simulink model "KD_cl_harness_forthao_breach"  (R2015a)
settings: Solver=ode45  StartTime=0  StopTime=50  FixedStep=0.01  MaxStep=0.005  RelTol=1e-4  AbsTol=1e-4
InitFcn:
  | load KD_const_coeffs_0624
  | load pexhat_stuff
  | load expcon
  | load thr_ff_map
undefined symbols (not defined in the file): c_0, c_1, c_100, c_1000, c_10000, c_1000inv, c_100inv, c_1_int, c_1d2p4, c_1p7, c_4400inv, c_5500inv, c_80, c_90, c_cal_phi, c_compmap, c_ctok, c_fflow_max, c_fflow_min, c_filt, c_flowdiv, c_flowmin, c_flowmult, c_inf, c_km1d2k, c_mm3tokgpers, c_n1, c_p00001, c_p01, c_p016, c_p1429, c_p1e9, c_p4167, c_p4d1p4, c_p5401, c_p9, c_pincomp, c_ra, c_rair, c_Rby1000, c_roacorr, c_rpmtoradpers, c_svrthrottle1, c_svrthrottle2, c_svrthrottlearg, c_svrthrottlebeta, c_ta_max, c_ta_min, c_V, c_vnliftmax, c_vnliftmin, Coefs, const, const_exhat, eegr_map, egrr_delay_init, epim_map, eplufin_ff_map, expcon, invta ... (+17)
libraries: simulink x5
(part 3 of 5)

== system KD_cl_harness_forthao_breach/ctrl_rb_explicit_20131031_v2/While_Iterator_Subsystem ==
  In1 : Inport
  In2 : Inport  Port=2
  In3 : Inport  Port=3
  In4 : Inport  Port=4
  In5 : Inport  Port=5
  In6 : Inport  Port=6
  In7 : Inport  Port=7
  In8 : Inport  Port=8
  pexz : Inport  Port=9
  Constant10 : Constant  Value=SVR_EGR_exhat.Beta
  Constant11 : Constant  Value=SVR_EGR_exhat.SV2
  Constant12 : Constant  Value=SVR_EGR_exhat.SV1
  Constant13 : Constant  Value=const_exhat.k
  Constant14 : Constant  Value=SVR_EGR_exhat.arg
  Constant7 : Constant  Value=const_exhat.Pcab
  Constant8 : Constant  Value=const_exhat.Tcab
  Gain10 : Gain  Gain=c_p01
      settings: AttributesFormatString=%<Gain>
  Gain11 : Gain  Gain=c_4400inv
      settings: AttributesFormatString=%<Gain>
  Mux14 : Mux  Inputs=2
  Saturation4 : Saturate  UpperLimit=c_inf  LowerLimit=c_80
      settings: AttributesFormatString=%<LowerLimit>\n%<UpperLimit>
  Saturation_Dynamic2 : simulink/Discontinuities/Saturation Dynamic  OutMin=[]  OutMax=[]  OutDataTypeStr=Inherit: Same as second input  OutDataType=fixdt(1, 16)  OutScaling=2^-10  DoSatur=off
  Sum14 : Sum  Inputs=++|
  While Iterator : WhileIterator
  newton : Subsystem
  pexmax1 : Constant  Value=1000  OutDataTypeStr=single  SampleTime=-1
      settings: AttributesFormatString=%<Value>\n%<SampleTime>
  unity2 : Constant  OutDataTypeStr=single  SampleTime=-1
      settings: AttributesFormatString=%<Value>\n%<SampleTime>
  y_cons4 : Constant  OutDataTypeStr=boolean  SampleTime=-1
      settings: AttributesFormatString=%<Value>\n%<SampleTime>
  Out1 : Outport
  Out2 : Outport  Port=2
  Out3 : Outport  Port=3
  wires:
  y_cons4/1 -> While Iterator/1
  Constant14/1 -> newton/5(arg)
  Constant12/1 -> newton/3(SV1)
  Constant10/1 -> newton/2(Beta)
  Gain11/1 -> Mux14/2
  Gain10/1 -> Mux14/1
  Mux14/1 -> newton/1(u)
  Constant7/1 -> newton/9(pcab)
  Constant8/1 -> newton/10(tcab)
  Constant13/1 -> newton/12(k)
  newton/1(pexkp1) -> Out1/1, Saturation_Dynamic2/2
  Saturation_Dynamic2/1 -> Out3/1
  unity2/1 -> Sum14/1
  Sum14/1 -> Saturation_Dynamic2/3
  pexmax1/1 -> Saturation_Dynamic2/1
  Constant11/1 -> newton/4(SV2)
  Saturation4/1 -> Sum14/2
  In1/1 -> Gain10/1
  In2/1 -> Gain11/1
  In3/1 -> newton/7(pin)
  In4/1 -> newton/8(wegrmeas)
  newton/2(dwdp) -> Out2/1
  In5/1 -> newton/11(tex)
  In6/1 -> newton/13(pex_ecu)
  In7/1 -> Saturation4/1
  In8/1 -> While Iterator/2
  pexz/1 -> newton/6(pex)

== system KD_cl_harness_forthao_breach/ctrl_rb_explicit_20131031_v2/custom_filter ==
  Input : Inport
  Data Store Read1 : DataStoreRead  DataStoreName=man_tuneFiltalpha  SampleTime=sample_time
  Data Store Read8 : DataStoreRead  DataStoreName=man_tuneFiltalpha  SampleTime=sample_time
  Delay1 : Delay  DelayLength=1  InitialCondition=0
  Product1 : Product  Inputs=**  RndMeth=Zero
  Product2 : Product  Inputs=**  RndMeth=Zero
  Saturation1 : Saturate  UpperLimit=1  LowerLimit=0
      settings: AttributesFormatString=%<LowerLimit>\n%<UpperLimit>
  Saturation4 : Saturate  UpperLimit=1  LowerLimit=0
      settings: AttributesFormatString=%<LowerLimit>\n%<UpperLimit>
  Sum1 : Sum  Inputs=+-|
  Sum11 : Sum  Inputs=++|
  man_tuneFiltalpha : Gain
  man_tuneFiltalpha1 : Gain
  zero1 : Constant  OutDataTypeStr=single  SampleTime=sample_time
      settings: AttributesFormatString=%<Value>\n%<SampleTime>
  Output : Outport  OutDataTypeStr=single
  wires:
  man_tuneFiltalpha1/1 -> Saturation1/1
  man_tuneFiltalpha/1 -> Saturation4/1
  Input/1 -> Product1/2
  Delay1/1 -> Product2/1
  Data Store Read8/1 -> man_tuneFiltalpha1/1
  Product2/1 -> Sum11/1
  Sum1/1 -> Product1/1
  Data Store Read1/1 -> man_tuneFiltalpha/1
  Saturation4/1 -> Sum1/2
  Saturation1/1 -> Product2/2
  Product1/1 -> Sum11/2
  zero1/1 -> Sum1/1
  Sum11/1 -> Output/1, Delay1/1

== system KD_cl_harness_forthao_breach/ctrl_rb_explicit_20131031_v2/custom_filter1 ==
  Input : Inport
  Data Store Read1 : DataStoreRead  DataStoreName=man_tuneFiltalpha  SampleTime=sample_time
  Data Store Read8 : DataStoreRead  DataStoreName=man_tuneFiltalpha  SampleTime=sample_time
  Delay1 : Delay  DelayLength=1  InitialCondition=0
  Product1 : Product  Inputs=**  RndMeth=Zero
  Product2 : Product  Inputs=**  RndMeth=Zero
  Saturation1 : Saturate  UpperLimit=1  LowerLimit=0
      settings: AttributesFormatString=%<LowerLimit>\n%<UpperLimit>
  Saturation4 : Saturate  UpperLimit=1  LowerLimit=0
      settings: AttributesFormatString=%<LowerLimit>\n%<UpperLimit>
  Sum1 : Sum  Inputs=+-|
  Sum11 : Sum  Inputs=++|
  man_tuneFiltalpha : Gain
  man_tuneFiltalpha1 : Gain
  zero1 : Constant  OutDataTypeStr=single  SampleTime=sample_time
      settings: AttributesFormatString=%<Value>\n%<SampleTime>
  Output : Outport  OutDataTypeStr=single
  wires:
  man_tuneFiltalpha1/1 -> Saturation1/1
  man_tuneFiltalpha/1 -> Saturation4/1
  Sum11/1 -> Delay1/1, Output/1
  zero1/1 -> Sum1/1
  Product1/1 -> Sum11/2
  Saturation1/1 -> Product2/2
  Saturation4/1 -> Sum1/2
  Data Store Read1/1 -> man_tuneFiltalpha/1
  Sum1/1 -> Product1/1
  Product2/1 -> Sum11/1
  Data Store Read8/1 -> man_tuneFiltalpha1/1
  Delay1/1 -> Product2/1
  Input/1 -> Product1/2

== system KD_cl_harness_forthao_breach/ctrl_rb_explicit_20131031_v2/custom_filter2 ==
  Input : Inport
  Data Store Read1 : DataStoreRead  DataStoreName=man_tuneFiltalpha  SampleTime=sample_time
  Data Store Read8 : DataStoreRead  DataStoreName=man_tuneFiltalpha  SampleTime=sample_time
  Delay1 : Delay  DelayLength=1  InitialCondition=0
  Product1 : Product  Inputs=**  RndMeth=Zero
  Product2 : Product  Inputs=**  RndMeth=Zero
  Saturation1 : Saturate  UpperLimit=1  LowerLimit=0
      settings: AttributesFormatString=%<LowerLimit>\n%<UpperLimit>
  Saturation4 : Saturate  UpperLimit=1  LowerLimit=0
      settings: AttributesFormatString=%<LowerLimit>\n%<UpperLimit>
  Sum1 : Sum  Inputs=+-|
  Sum11 : Sum  Inputs=++|
  man_tuneFiltalpha : Gain
  man_tuneFiltalpha1 : Gain
  zero1 : Constant  OutDataTypeStr=single  SampleTime=sample_time
      settings: AttributesFormatString=%<Value>\n%<SampleTime>
  Output : Outport  OutDataTypeStr=single
  wires:
  man_tuneFiltalpha1/1 -> Saturation1/1
  man_tuneFiltalpha/1 -> Saturation4/1
  Sum11/1 -> Delay1/1, Output/1
  zero1/1 -> Sum1/1
  Product1/1 -> Sum11/2
  Saturation1/1 -> Product2/2
  Saturation4/1 -> Sum1/2
  Data Store Read1/1 -> man_tuneFiltalpha/1
  Sum1/1 -> Product1/1
  Product2/1 -> Sum11/1
  Data Store Read8/1 -> man_tuneFiltalpha1/1
  Delay1/1 -> Product2/1
  Input/1 -> Product1/2

== system KD_cl_harness_forthao_breach/ctrl_rb_explicit_20131031_v2/custom_filter3 ==
  Input : Inport
  Data Store Read1 : DataStoreRead  DataStoreName=man_tuneFiltalpha  SampleTime=sample_time
  Data Store Read8 : DataStoreRead  DataStoreName=man_tuneFiltalpha  SampleTime=sample_time
  Delay1 : Delay  DelayLength=1  InitialCondition=0
  Product1 : Product  Inputs=**  RndMeth=Zero
  Product2 : Product  Inputs=**  RndMeth=Zero
  Saturation1 : Saturate  UpperLimit=1  LowerLimit=0
      settings: AttributesFormatString=%<LowerLimit>\n%<UpperLimit>
  Saturation4 : Saturate  UpperLimit=1  LowerLimit=0
      settings: AttributesFormatString=%<LowerLimit>\n%<UpperLimit>
  Sum1 : Sum  Inputs=+-|
  Sum11 : Sum  Inputs=++|
  man_tuneFiltalpha : Gain
  man_tuneFiltalpha1 : Gain
  zero1 : Constant  OutDataTypeStr=single  SampleTime=sample_time
      settings: AttributesFormatString=%<Value>\n%<SampleTime>
  Output : Outport  OutDataTypeStr=single
  wires:
  man_tuneFiltalpha1/1 -> Saturation1/1
  man_tuneFiltalpha/1 -> Saturation4/1
  Input/1 -> Product1/2
  Delay1/1 -> Product2/1
  Data Store Read8/1 -> man_tuneFiltalpha1/1
  Product2/1 -> Sum11/1
  Sum1/1 -> Product1/1
  Data Store Read1/1 -> man_tuneFiltalpha/1
  Saturation4/1 -> Sum1/2
  Saturation1/1 -> Product2/2
  Product1/1 -> Sum11/2
  zero1/1 -> Sum1/1
  Sum11/1 -> Output/1, Delay1/1

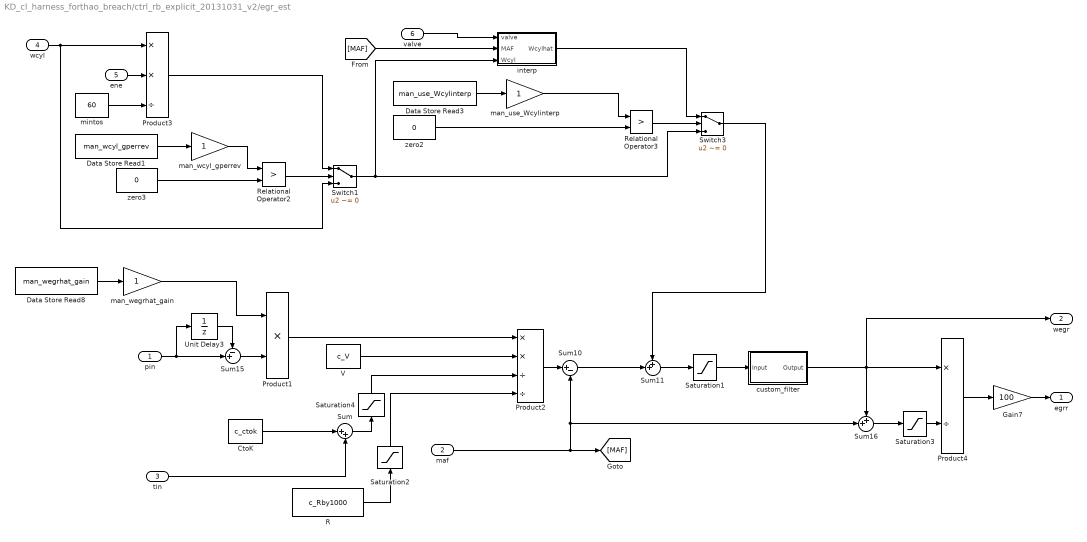
== system KD_cl_harness_forthao_breach/ctrl_rb_explicit_20131031_v2/egr_est ==
  pin : Inport
  maf : Inport  Port=2
  tin : Inport  Port=3
  wcyl : Inport  Port=4
  ene : Inport  Port=5
  valve : Inport  Port=6
  CtoK : Constant  Value=c_ctok  OutDataTypeStr=single
      settings: AttributesFormatString=%<Value>
  Data Store Read1 : DataStoreRead  DataStoreName=man_wcyl_gperrev  SampleTime=sample_time
  Data Store Read3 : DataStoreRead  DataStoreName=man_use_Wcylinterp  SampleTime=sample_time
  Data Store Read8 : DataStoreRead  DataStoreName=man_wegrhat_gain  SampleTime=sample_time
  Gain7 : Gain  Gain=100
      settings: AttributesFormatString=%<Gain>
  Product1 : Product  Inputs=**  RndMeth=Zero
  Product2 : Product  Inputs=**//  RndMeth=Zero
  Product3 : Product  Inputs=**/  RndMeth=Zero
  Product4 : Product  Inputs=*/  RndMeth=Zero
  R : Constant  Value=c_Rby1000  OutDataTypeStr=single
      settings: AttributesFormatString=%<Value>
  Relational Operator2 : RelationalOperator  Operator=>  OutDataTypeStr=boolean
      settings: AttributesFormatString=%<Operator>
  Relational Operator3 : RelationalOperator  Operator=>  OutDataTypeStr=boolean
      settings: AttributesFormatString=%<Operator>
  Saturation1 : Saturate  UpperLimit=c_inf  LowerLimit=c_0
      settings: AttributesFormatString=%<LowerLimit>\n%<UpperLimit>
  Saturation2 : Saturate  UpperLimit=c_inf  LowerLimit=c_p1e9
      settings: AttributesFormatString=%<LowerLimit>\n%<UpperLimit>
  Saturation3 : Saturate  UpperLimit=c_inf  LowerLimit=c_p00001
      settings: AttributesFormatString=%<LowerLimit>\n%<UpperLimit>
  Saturation4 : Saturate  UpperLimit=c_inf  LowerLimit=c_p1e9
      settings: AttributesFormatString=%<LowerLimit>\n%<UpperLimit>
  Sum : Sum  Inputs=|++
  Sum10 : Sum  Inputs=|+-
  Sum11 : Sum  Inputs=++|
  Sum15 : Sum  Inputs=-+|
  Sum16 : Sum  Inputs=++|
  Switch1 : Switch  Criteria=u2 ~= 0
      settings: AttributesFormatString=%<Criteria>
  Switch3 : Switch  Criteria=u2 ~= 0
      settings: AttributesFormatString=%<Criteria>
  Unit Delay3 : UnitDelay  SampleTime=-1
  V : Constant  Value=c_V  OutDataTypeStr=single
      settings: AttributesFormatString=%<Value>
  custom_filter : Subsystem  Tag=FilterWizardSubSystem
      settings: ErrorFcn=dspFilterRealizedInBasicElemsAlgLoopErrFcnCallback
  interp : Subsystem  Tag=FilterWizardSubSystem
      settings: ErrorFcn=dspFilterRealizedInBasicElemsAlgLoopErrFcnCallback
  man_use_Wcylinterp : Gain
  man_wcyl_gperrev : Gain
  man_wegrhat_gain : Gain
  mintos : Constant  Value=60  OutDataTypeStr=single
      settings: AttributesFormatString=%<Value>
  zero2 : Constant  Value=0  OutDataTypeStr=single  SampleTime=sample_time
      settings: AttributesFormatString=%<Value>\n%<SampleTime>
  zero3 : Constant  Value=0  OutDataTypeStr=single  SampleTime=sample_time
      settings: AttributesFormatString=%<Value>\n%<SampleTime>
  egrr : Outport
  wegr : Outport  Port=2
  wires:
  Switch1/1 -> Switch3/3, interp/3(Wcyl)
  Product3/1 -> Switch1/1
  Data Store Read1/1 -> man_wcyl_gperrev/1
  Relational Operator2/1 -> Switch1/2
  zero3/1 -> Relational Operator2/2
  Saturation4/1 -> Product2/3
  Saturation2/1 -> Product2/4
  CtoK/1 -> Sum/1
  V/1 -> Product2/2
  Sum/1 -> Saturation4/1
  R/1 -> Saturation2/1
  Product2/1 -> Sum10/1
  pin/1 -> Unit Delay3/1, Sum15/2
  Sum15/1 -> Product1/2
  Product1/1 -> Product2/1
  Unit Delay3/1 -> Sum15/1
  mintos/1 -> Product3/3
  Sum11/1 -> Saturation1/1
  Sum16/1 -> Saturation3/1
  Product4/1 -> Gain7/1
  Gain7/1 -> egrr/1
  maf/1 -> Sum10/2, Sum16/2, [MAF]
  tin/1 -> Sum/2
  wcyl/1 -> Switch1/3, Product3/1
  ene/1 -> Product3/2
  Sum10/1 -> Sum11/2
  Data Store Read8/1 -> man_wegrhat_gain/1
  Saturation1/1 -> custom_filter/1(Input)
  Saturation3/1 -> Product4/2
  Data Store Read3/1 -> man_use_Wcylinterp/1
  Relational Operator3/1 -> Switch3/2
  zero2/1 -> Relational Operator3/2
  Switch3/1 -> Sum11/1
  interp/1(Wcylhat) -> Switch3/1
  [MAF] -> interp/2(MAF)
  valve/1 -> interp/1(valve)
  custom_filter/1(Output) -> Product4/1, Sum16/1, wegr/1
  man_wegrhat_gain/1 -> Product1/1
  man_wcyl_gperrev/1 -> Relational Operator2/1
  man_use_Wcylinterp/1 -> Relational Operator3/1

== system KD_cl_harness_forthao_breach/ctrl_rb_explicit_20131031_v2/expcon ==
  u : Inport
  Terminator1 : Terminator
  find_region : Subsystem
  get_ctrl : Subsystem
  u_star : Outport
  region_num : Outport  Port=2
  wires:
  find_region/2(rv) -> Terminator1/1
  find_region/1(region) -> get_ctrl/1(region), region_num/1
  [u] -> find_region/1(u)
  [u] -> get_ctrl/2(u)
  u/1 -> [u]
  get_ctrl/1(u_star) -> u_star/1

== system KD_cl_harness_forthao_breach/ctrl_rb_explicit_20131031_v2/invert_flow ==
  valve_flow_command : Inport
  intake_pressure : Inport  Port=2
  exhuast_pressure : Inport  Port=3
  Tintake : Inport  Port=4
  ne_rpm : Inport  Port=5
  Gain : Gain  Gain=c_1000
  Gain1 : Gain  Gain=c_1000
  Product1 : Product  Inputs=*//  SaturateOnIntegerOverflow=on  RndMeth=Zero  InputSameDT=on  OutDataTypeStr=Inherit: Same as first input
  Ra : Constant  Value=c_ra  OutDataTypeStr=single
  Saturation1 : Saturate  UpperLimit=c_80  LowerLimit=c_0
      settings: AttributesFormatString=%<LowerLimit>\n%<UpperLimit>
  Saturation4 : Saturate  UpperLimit=c_ta_max  LowerLimit=c_ta_min
      settings: AttributesFormatString=%<LowerLimit>\n%<UpperLimit>
  valve_inversion : Subsystem
  uvalve : Outport
  wires:
  ne_rpm/1 -> valve_inversion/5(ne_rpm)
  Saturation1/1 -> uvalve/1
  valve_inversion/1(valve_angle) -> Saturation1/1
  Gain1/1 -> valve_inversion/3(pintake)
  Gain/1 -> Product1/1, valve_inversion/2(pexhaust)
  Ra/1 -> Product1/3
  Product1/1 -> valve_inversion/1(Ro_a)
  exhuast_pressure/1 -> Gain/1
  intake_pressure/1 -> Gain1/1
  valve_flow_command/1 -> valve_inversion/4(uwegr)
  Tintake/1 -> [Tin]
  [Tin] -> Saturation4/1
  Saturation4/1 -> Product1/2

== system KD_cl_harness_forthao_breach/ctrl_rb_explicit_20131031_v2/ntestimator ==
  u_EGR_throttle : Inport
  omega_engine_rpm : Inport  Port=2
  p_intake_man : Inport  Port=3
  T_out_IC : Inport  Port=4
  maf : Inport  Port=5
  Data Store Write25 : DataStoreWrite  DataStoreName=mon_pthr
  Divide : Product  Inputs=/*
  Gain : Gain  Gain=1000
      settings: AttributesFormatString=%<Gain>
  Lookup_Table_2D : Lookup2D  RowIndex=c_vwcompdes  ColumnIndex=c_vpout  Table=c_compmap
  Throttle_Model : Subsystem
  conversion to radpers : Gain  Gain=c_rpmtoradpers
  custom_filter : Subsystem  Tag=FilterWizardSubSystem
      settings: ErrorFcn=dspFilterRealizedInBasicElemsAlgLoopErrFcnCallback
  mon_pthr : Gain
  pincomp : Constant  Value=c_pincomp  OutDataTypeStr=single  SampleTime=sample_time
      settings: AttributesFormatString=%<Value>\n%<SampleTime>
  ntest : Outport
  wires:
  p_intake_man/1 -> Gain/1
  Throttle_Model/1(p_pre_throttle) -> Divide/2, mon_pthr/1
  maf/1 -> custom_filter/1(Input), [maf]
  pincomp/1 -> Divide/1
  Divide/1 -> Lookup_Table_2D/2
  [maf] -> Lookup_Table_2D/1
  Lookup_Table_2D/1 -> conversion to radpers/1
  conversion to radpers/1 -> ntest/1
  u_EGR_throttle/1 -> Throttle_Model/1(TA_deg)
  omega_engine_rpm/1 -> Throttle_Model/2(Ne_rpm)
  Gain/1 -> Throttle_Model/3(Pim_Pa)
  T_out_IC/1 -> Throttle_Model/4(Tam_K)
  custom_filter/1(Output) -> Throttle_Model/5(wegrthr)
  mon_pthr/1 -> Data Store Write25/1

== system KD_cl_harness_forthao_breach/ctrl_rb_explicit_20131031_v2/obs ==
  map : Inport
  egrr : Inport  Port=2
  xhat : Inport  Port=3
  delu : Inport  Port=4
  Gain : Gain  Gain=expcon.obsC  Multiplication=Matrix(K*u) (u vector)
      settings: AttributesFormatString=%<Multiplication>
  Gain1 : Gain  Gain=expcon.obsL  Multiplication=Matrix(K*u) (u vector)
      settings: AttributesFormatString=%<Multiplication>
  Gain2 : Gain  Gain=expcon.obsA  Multiplication=Matrix(K*u) (u vector)
      settings: AttributesFormatString=%<Multiplication>
  Gain3 : Gain  Gain=expcon.obsB  Multiplication=Matrix(K*u) (u vector)
      settings: AttributesFormatString=%<Multiplication>
  Mux : Mux  Inputs=2
  Sum : Sum  Inputs=++|
  Sum1 : Sum  Inputs=|+-
  Sum2 : Sum  Inputs=|++
  Unit Delay : UnitDelay  InitialCondition=map_delay_init  SampleTime=-1
      settings: AttributesFormatString=%<X0>
  Unit Delay1 : UnitDelay  InitialCondition=egrr_delay_init  SampleTime=-1
      settings: AttributesFormatString=%<X0>
  xhatp : Outport
  wires:
  Unit Delay/1 -> Mux/1
  Unit Delay1/1 -> Mux/2
  delu/1 -> Gain3/1
  Gain2/1 -> Sum/2
  Gain1/1 -> Sum/1
  Sum1/1 -> Gain1/1
  Gain/1 -> Sum1/2
  Mux/1 -> Sum1/1
  egrr/1 -> Unit Delay1/1
  map/1 -> Unit Delay/1
  xhat/1 -> Gain2/1, Gain/1
  Sum/1 -> Sum2/1
  Sum2/1 -> xhatp/1
  Gain3/1 -> Sum2/2

== system KD_cl_harness_forthao_breach/ctrl_rb_explicit_20131031_v2/reduced_obs ==
  map : Inport
  egrr : Inport  Port=2
  xhatROpm1 : Inport  Port=3
  u : Inport  Port=4
  Gain : Gain  Gain=expcon.RobsC  Multiplication=Matrix(K*u) (u vector)
      settings: AttributesFormatString=%<Multiplication>
  Gain1 : Gain  Gain=expcon.RobsL  Multiplication=Matrix(K*u) (u vector)
      settings: AttributesFormatString=%<Multiplication>
  Gain2 : Gain  Gain=expcon.RobsA  Multiplication=Matrix(K*u) (u vector)
      settings: AttributesFormatString=%<Multiplication>
  Gain3 : Gain  Gain=expcon.RobsB  Multiplication=Matrix(K*u) (u vector)
      settings: AttributesFormatString=%<Multiplication>
  Gain4 : Gain  Gain=expcon.RobsD  Multiplication=Matrix(K*u) (u vector)
      settings: AttributesFormatString=%<Multiplication>
  Mux : Mux  Inputs=2
  Mux1 : Mux  Inputs=3
  Sum : Sum  Inputs=++|
  Sum1 : Sum  Inputs=-+-
  Sum2 : Sum  Inputs=|++
  Sum3 : Sum  Inputs=-+|
  Sum4 : Sum  Inputs=-+|
  Sum5 : Sum  Inputs=|+-
  Unit Delay1 : UnitDelay  SampleTime=-1
      settings: AttributesFormatString=%<X0>
  Unit Delay2 : UnitDelay  SampleTime=-1
      settings: AttributesFormatString=%<X0>
  Unit Delay5 : UnitDelay  SampleTime=-1
      settings: AttributesFormatString=%<X0>
  ue : Constant  Value=expcon.Robsue  OutDataTypeStr=single  SampleTime=sample_time
      settings: AttributesFormatString=%<Value>\n%<SampleTime>
  ye : Constant  Value=expcon.Robsye  OutDataTypeStr=single  SampleTime=sample_time
      settings: AttributesFormatString=%<Value>\n%<SampleTime>
  xhatRO : Outport  OutDataTypeStr=single
  xhat : Outport  Port=2
  delxhat : Outport  Port=3
  wires:
  Gain3/1 -> Sum2/2
  Sum/1 -> Sum2/1
  xhatROpm1/1 -> Gain/1, Gain2/1
  map/1 -> Mux/1, [map]
  egrr/1 -> Mux/2, [egrr]
  Sum1/1 -> Gain1/1
  Gain1/1 -> Sum/1
  Gain2/1 -> Sum/2
  Gain/1 -> Sum1/3
  ye/1 -> Sum1/1
  u/1 -> Sum3/2
  Sum3/1 -> Gain3/1, Gain4/1
  ue/1 -> Sum3/1
  Mux/1 -> Sum4/2
  Sum4/1 -> Sum1/2
  Gain4/1 -> Sum4/1
  Sum2/1 -> Sum5/1, Unit Delay5/1, xhatRO/1
  Unit Delay5/1 -> Sum5/2
  Sum5/1 -> Mux1/1, delxhat/1
  Mux1/1 -> xhat/1
  Unit Delay1/1 -> Mux1/2
  Unit Delay2/1 -> Mux1/3
  [map] -> Unit Delay1/1
  [egrr] -> Unit Delay2/1

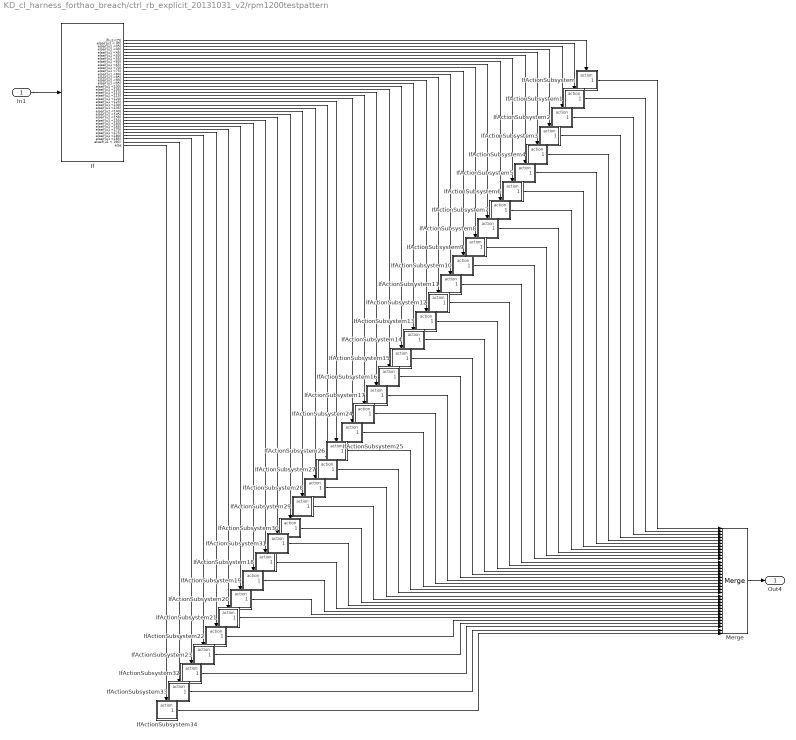
== system KD_cl_harness_forthao_breach/ctrl_rb_explicit_20131031_v2/rpm1200testpattern ==
  In1 : Inport  OutDataTypeStr=single
  If : If  IfExpression=u1<25  ElseIfExpressions=u1 < 30, u1 <35, u1 <40, u1 <45, u1 <50, u1 <55, u1 <60, u1 <65, u1 <70, u1 <75, u1 <80, u1 <85, u1 <90, u1 <95, u1 <100, u1 <105, u1 <110, u1 <115, u1 <120, u1 <125, u1 <130, u1 <135, u1 <140, u1 <145, u1 <150, u1 <155, u1 <160, u1 <165, u1 <170, u1 <175, u1 <180, u1 <185 ,u1 < 190
  IfActionSubsystem : Subsystem  TreatAsAtomicUnit=on
  IfActionSubsystem1 : Subsystem  TreatAsAtomicUnit=on
  IfActionSubsystem10 : Subsystem  TreatAsAtomicUnit=on
  IfActionSubsystem11 : Subsystem  TreatAsAtomicUnit=on
  IfActionSubsystem12 : Subsystem  TreatAsAtomicUnit=on
  IfActionSubsystem13 : Subsystem  TreatAsAtomicUnit=on
  IfActionSubsystem14 : Subsystem  TreatAsAtomicUnit=on
  IfActionSubsystem15 : Subsystem  TreatAsAtomicUnit=on
  IfActionSubsystem16 : Subsystem  TreatAsAtomicUnit=on
  IfActionSubsystem17 : Subsystem  TreatAsAtomicUnit=on
  IfActionSubsystem18 : Subsystem  TreatAsAtomicUnit=on
  IfActionSubsystem19 : Subsystem  TreatAsAtomicUnit=on
  IfActionSubsystem2 : Subsystem  TreatAsAtomicUnit=on
  IfActionSubsystem20 : Subsystem  TreatAsAtomicUnit=on
  IfActionSubsystem21 : Subsystem  TreatAsAtomicUnit=on
  IfActionSubsystem22 : Subsystem  TreatAsAtomicUnit=on
  IfActionSubsystem23 : Subsystem  TreatAsAtomicUnit=on
  IfActionSubsystem24 : Subsystem  TreatAsAtomicUnit=on
  IfActionSubsystem25 : Subsystem  TreatAsAtomicUnit=on
  IfActionSubsystem26 : Subsystem  TreatAsAtomicUnit=on
  IfActionSubsystem27 : Subsystem  TreatAsAtomicUnit=on
  IfActionSubsystem28 : Subsystem  TreatAsAtomicUnit=on
  IfActionSubsystem29 : Subsystem  TreatAsAtomicUnit=on
  IfActionSubsystem3 : Subsystem  TreatAsAtomicUnit=on
  IfActionSubsystem30 : Subsystem  TreatAsAtomicUnit=on
  IfActionSubsystem31 : Subsystem  TreatAsAtomicUnit=on
  IfActionSubsystem32 : Subsystem  TreatAsAtomicUnit=on
  IfActionSubsystem33 : Subsystem  TreatAsAtomicUnit=on
  IfActionSubsystem34 : Subsystem  TreatAsAtomicUnit=on
  IfActionSubsystem4 : Subsystem  TreatAsAtomicUnit=on
  IfActionSubsystem5 : Subsystem  TreatAsAtomicUnit=on
  IfActionSubsystem6 : Subsystem  TreatAsAtomicUnit=on
  IfActionSubsystem7 : Subsystem  TreatAsAtomicUnit=on
  IfActionSubsystem8 : Subsystem  TreatAsAtomicUnit=on
  IfActionSubsystem9 : Subsystem  TreatAsAtomicUnit=on
  Merge : Merge  Inputs=35  InitialOutput=[150;50;150]
      settings: AttributesFormatString=%<InitialOutput>
  Out4 : Outport  OutDataTypeStr=single
  wires:
  IfActionSubsystem32/1(Out1) -> Merge/33
  IfActionSubsystem23/1(Out1) -> Merge/32
  IfActionSubsystem22/1(Out1) -> Merge/31
  If/32 -> IfActionSubsystem23/Action
  If/31 -> IfActionSubsystem22/Action
  Merge/1 -> Out4/1
  In1/1 -> If/1
  IfActionSubsystem21/1(Out1) -> Merge/30
  IfActionSubsystem20/1(Out1) -> Merge/29
  IfActionSubsystem19/1(Out1) -> Merge/28
  IfActionSubsystem18/1(Out1) -> Merge/27
  IfActionSubsystem31/1(Out1) -> Merge/26
  IfActionSubsystem30/1(Out1) -> Merge/25
  IfActionSubsystem29/1(Out1) -> Merge/24
  IfActionSubsystem28/1(Out1) -> Merge/23
  IfActionSubsystem27/1(Out1) -> Merge/22
  IfActionSubsystem26/1(Out1) -> Merge/21
  IfActionSubsystem25/1(Out1) -> Merge/20
  IfActionSubsystem24/1(Out1) -> Merge/19
  IfActionSubsystem17/1(Out1) -> Merge/18
  IfActionSubsystem16/1(Out1) -> Merge/17
  IfActionSubsystem15/1(Out1) -> Merge/16
  IfActionSubsystem14/1(Out1) -> Merge/15
  IfActionSubsystem13/1(Out1) -> Merge/14
  IfActionSubsystem12/1(Out1) -> Merge/13
  IfActionSubsystem11/1(Out1) -> Merge/12
  IfActionSubsystem10/1(Out1) -> Merge/11
  IfActionSubsystem9/1(Out1) -> Merge/10
  IfActionSubsystem8/1(Out1) -> Merge/9
  IfActionSubsystem7/1(Out1) -> Merge/8
  IfActionSubsystem6/1(Out1) -> Merge/7
  IfActionSubsystem5/1(Out1) -> Merge/6
  IfActionSubsystem4/1(Out1) -> Merge/5
  IfActionSubsystem3/1(Out1) -> Merge/4
  IfActionSubsystem2/1(Out1) -> Merge/3
  IfActionSubsystem1/1(Out1) -> Merge/2
  IfActionSubsystem/1(Out1) -> Merge/1
  If/30 -> IfActionSubsystem21/Action
  If/29 -> IfActionSubsystem20/Action
  If/28 -> IfActionSubsystem19/Action
  If/27 -> IfActionSubsystem18/Action
  If/26 -> IfActionSubsystem31/Action
  If/25 -> IfActionSubsystem30/Action
  If/24 -> IfActionSubsystem29/Action
  If/23 -> IfActionSubsystem28/Action
  If/22 -> IfActionSubsystem27/Action
  If/21 -> IfActionSubsystem26/Action
  If/20 -> IfActionSubsystem25/Action
  If/19 -> IfActionSubsystem24/Action
  If/18 -> IfActionSubsystem17/Action
  If/17 -> IfActionSubsystem16/Action
  If/16 -> IfActionSubsystem15/Action
  If/15 -> IfActionSubsystem14/Action
  If/14 -> IfActionSubsystem13/Action
  If/13 -> IfActionSubsystem12/Action
  If/12 -> IfActionSubsystem11/Action
  If/11 -> IfActionSubsystem10/Action
  If/10 -> IfActionSubsystem9/Action
  If/9 -> IfActionSubsystem8/Action
  If/8 -> IfActionSubsystem7/Action
  If/7 -> IfActionSubsystem6/Action
  If/6 -> IfActionSubsystem5/Action
  If/5 -> IfActionSubsystem4/Action
  If/4 -> IfActionSubsystem3/Action
  If/3 -> IfActionSubsystem2/Action
  If/2 -> IfActionSubsystem1/Action
  If/1 -> IfActionSubsystem/Action
  If/33 -> IfActionSubsystem32/Action
  If/34 -> IfActionSubsystem33/Action
  If/35 -> IfActionSubsystem34/Action
  IfActionSubsystem33/1(Out1) -> Merge/34
  IfActionSubsystem34/1(Out1) -> Merge/35

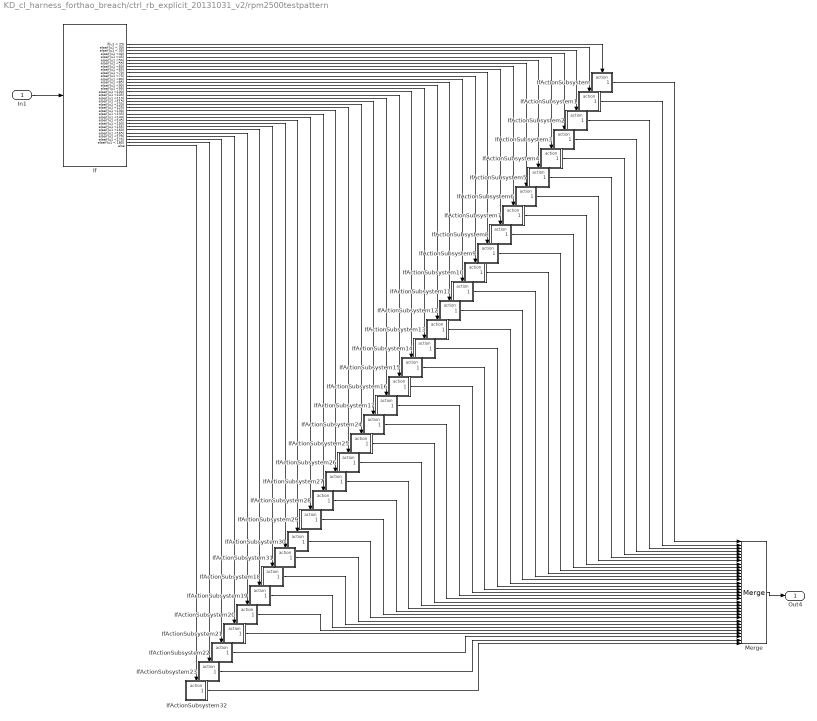
== system KD_cl_harness_forthao_breach/ctrl_rb_explicit_20131031_v2/rpm2500testpattern ==
  In1 : Inport  OutDataTypeStr=single
  If : If  IfExpression=u1 < 25  ElseIfExpressions=u1 < 30, u1 < 35, u1 <40, u1 <45, u1 <50, u1 <55, u1 <60, u1 <65, u1 <70, u1 <75, u1 <80, u1 <85, u1 <90, u1 <95, u1 <100, u1 <105, u1 <110, u1 <115, u1 <120, u1 <125, u1 <130, u1 <135, u1 <140, u1 <145, u1 <150, u1 <155, u1 <160, u1 <165, u1 <170, u1 <175 , u1 < 180
  IfActionSubsystem : Subsystem  TreatAsAtomicUnit=on
  IfActionSubsystem1 : Subsystem  TreatAsAtomicUnit=on
  IfActionSubsystem10 : Subsystem  TreatAsAtomicUnit=on
  IfActionSubsystem11 : Subsystem  TreatAsAtomicUnit=on
  IfActionSubsystem12 : Subsystem  TreatAsAtomicUnit=on
  IfActionSubsystem13 : Subsystem  TreatAsAtomicUnit=on
  IfActionSubsystem14 : Subsystem  TreatAsAtomicUnit=on
  IfActionSubsystem15 : Subsystem  TreatAsAtomicUnit=on
  IfActionSubsystem16 : Subsystem  TreatAsAtomicUnit=on
  IfActionSubsystem17 : Subsystem  TreatAsAtomicUnit=on
  IfActionSubsystem18 : Subsystem  TreatAsAtomicUnit=on
  IfActionSubsystem19 : Subsystem  TreatAsAtomicUnit=on
  IfActionSubsystem2 : Subsystem  TreatAsAtomicUnit=on
  IfActionSubsystem20 : Subsystem  TreatAsAtomicUnit=on
  IfActionSubsystem21 : Subsystem  TreatAsAtomicUnit=on
  IfActionSubsystem22 : Subsystem  TreatAsAtomicUnit=on
  IfActionSubsystem23 : Subsystem  TreatAsAtomicUnit=on
  IfActionSubsystem24 : Subsystem  TreatAsAtomicUnit=on
  IfActionSubsystem25 : Subsystem  TreatAsAtomicUnit=on
  IfActionSubsystem26 : Subsystem  TreatAsAtomicUnit=on
  IfActionSubsystem27 : Subsystem  TreatAsAtomicUnit=on
  IfActionSubsystem28 : Subsystem  TreatAsAtomicUnit=on
  IfActionSubsystem29 : Subsystem  TreatAsAtomicUnit=on
  IfActionSubsystem3 : Subsystem  TreatAsAtomicUnit=on
  IfActionSubsystem30 : Subsystem  TreatAsAtomicUnit=on
  IfActionSubsystem31 : Subsystem  TreatAsAtomicUnit=on
  IfActionSubsystem32 : Subsystem  TreatAsAtomicUnit=on
  IfActionSubsystem4 : Subsystem  TreatAsAtomicUnit=on
  IfActionSubsystem5 : Subsystem  TreatAsAtomicUnit=on
  IfActionSubsystem6 : Subsystem  TreatAsAtomicUnit=on
  IfActionSubsystem7 : Subsystem  TreatAsAtomicUnit=on
  IfActionSubsystem8 : Subsystem  TreatAsAtomicUnit=on
  IfActionSubsystem9 : Subsystem  TreatAsAtomicUnit=on
  Merge : Merge  Inputs=33  InitialOutput=[170;50;250]
      settings: AttributesFormatString=%<InitialOutput>
  Out4 : Outport  OutDataTypeStr=single
  wires:
  If/1 -> IfActionSubsystem/Action
  If/2 -> IfActionSubsystem1/Action
  If/3 -> IfActionSubsystem2/Action
  If/4 -> IfActionSubsystem3/Action
  If/5 -> IfActionSubsystem4/Action
  If/6 -> IfActionSubsystem5/Action
  If/7 -> IfActionSubsystem6/Action
  If/8 -> IfActionSubsystem7/Action
  If/9 -> IfActionSubsystem8/Action
  If/10 -> IfActionSubsystem9/Action
  If/11 -> IfActionSubsystem10/Action
  If/12 -> IfActionSubsystem11/Action
  If/13 -> IfActionSubsystem12/Action
  If/14 -> IfActionSubsystem13/Action
  If/15 -> IfActionSubsystem14/Action
  If/16 -> IfActionSubsystem15/Action
  If/17 -> IfActionSubsystem16/Action
  If/18 -> IfActionSubsystem17/Action
  If/19 -> IfActionSubsystem24/Action
  If/20 -> IfActionSubsystem25/Action
  If/21 -> IfActionSubsystem26/Action
  If/22 -> IfActionSubsystem27/Action
  If/23 -> IfActionSubsystem28/Action
  If/24 -> IfActionSubsystem29/Action
  If/25 -> IfActionSubsystem30/Action
  If/26 -> IfActionSubsystem31/Action
  If/27 -> IfActionSubsystem18/Action
  If/28 -> IfActionSubsystem19/Action
  If/29 -> IfActionSubsystem20/Action
  If/30 -> IfActionSubsystem21/Action
  IfActionSubsystem/1(Out1) -> Merge/1
  IfActionSubsystem1/1(Out1) -> Merge/2
  IfActionSubsystem2/1(Out1) -> Merge/3
  IfActionSubsystem3/1(Out1) -> Merge/4
  IfActionSubsystem4/1(Out1) -> Merge/5
  IfActionSubsystem5/1(Out1) -> Merge/6
  IfActionSubsystem6/1(Out1) -> Merge/7
  IfActionSubsystem7/1(Out1) -> Merge/8
  IfActionSubsystem8/1(Out1) -> Merge/9
  IfActionSubsystem9/1(Out1) -> Merge/10
  IfActionSubsystem10/1(Out1) -> Merge/11
  IfActionSubsystem11/1(Out1) -> Merge/12
  IfActionSubsystem12/1(Out1) -> Merge/13
  IfActionSubsystem13/1(Out1) -> Merge/14
  IfActionSubsystem14/1(Out1) -> Merge/15
  IfActionSubsystem15/1(Out1) -> Merge/16
  IfActionSubsystem16/1(Out1) -> Merge/17
  IfActionSubsystem17/1(Out1) -> Merge/18
  IfActionSubsystem24/1(Out1) -> Merge/19
  IfActionSubsystem25/1(Out1) -> Merge/20
  IfActionSubsystem26/1(Out1) -> Merge/21
  IfActionSubsystem27/1(Out1) -> Merge/22
  IfActionSubsystem28/1(Out1) -> Merge/23
  IfActionSubsystem29/1(Out1) -> Merge/24
  IfActionSubsystem30/1(Out1) -> Merge/25
  IfActionSubsystem31/1(Out1) -> Merge/26
  IfActionSubsystem18/1(Out1) -> Merge/27
  IfActionSubsystem19/1(Out1) -> Merge/28
  IfActionSubsystem20/1(Out1) -> Merge/29
  IfActionSubsystem21/1(Out1) -> Merge/30
  In1/1 -> If/1
  Merge/1 -> Out4/1
  If/31 -> IfActionSubsystem22/Action
  If/32 -> IfActionSubsystem23/Action
  If/33 -> IfActionSubsystem32/Action
  IfActionSubsystem22/1(Out1) -> Merge/31
  IfActionSubsystem23/1(Out1) -> Merge/32
  IfActionSubsystem32/1(Out1) -> Merge/33

== system KD_cl_harness_forthao_breach/ctrl_rb_explicit_20131031_v2/set_point_maps ==
  fuel_rate_mm3perst : Inport
  engine_speed_rpm : Inport  Port=2
  Data Store Read1 : DataStoreRead  DataStoreName=man_egrrefadd  SampleTime=sample_time
  Data Store Read3 : DataStoreRead  DataStoreName=man_pinrefadd  SampleTime=sample_time
  EGR_rate_map : Subsystem
  Saturation1 : Saturate  UpperLimit=c_inf  LowerLimit=c_0
      settings: AttributesFormatString=%<LowerLimit>\n%<UpperLimit>
  Sum2 : Sum  Inputs=|++
  Sum3 : Sum  Inputs=|++
  intake_pressure_map : Subsystem
  man_egrrefadd : Gain
  man_pinrefadd : Gain
  intake_pressure_ref : Outport
  EGR_ref : Outport  Port=2
  wires:
  [Ne] -> EGR_rate_map/2(engine_speed)
  [fuel_rate] -> EGR_rate_map/1(fuel_rate_mm3perst)
  fuel_rate_mm3perst/1 -> intake_pressure_map/1(fuel_rate_mm3perst), [fuel_rate]
  engine_speed_rpm/1 -> [Ne], intake_pressure_map/2(engine_speed)
  intake_pressure_map/1(intake_manifold_pressure_ref) -> Sum2/1
  Sum2/1 -> intake_pressure_ref/1
  EGR_rate_map/1(EGR_rate_ref) -> Sum3/1
  Sum3/1 -> Saturation1/1
  Saturation1/1 -> EGR_ref/1
  Data Store Read3/1 -> man_pinrefadd/1
  Data Store Read1/1 -> man_egrrefadd/1
  man_pinrefadd/1 -> Sum2/2
  man_egrrefadd/1 -> Sum3/2

== system KD_cl_harness_forthao_breach/pre-throttle manifold/p_preThrottle ==
  W_compressor : Inport
  W_throttle : Inport  Port=2
  T_out_compressor : Inport  Port=3
  T_out_IC_data : Inport  Port=4
  Cus_integrator : Subsystem
  Fcn1 : Fcn  Expr=u(4)*(u(1) - u(2))
  Mux : Mux
  gamma*R/V_preThrottle : Gain  Gain=const.gamma_air*const.R_specific_air_KJ_per_kg_kelvin/Coefs.V_prethrottle_m3
  "p_pre_throttle " : Outport
  wires:
  Cus_integrator/1(p_preThrottle) -> "p_pre_throttle "/1
  gamma*R/V_preThrottle/1 -> Cus_integrator/1(in)
  Fcn1/1 -> gamma*R/V_preThrottle/1
  Mux/1 -> Fcn1/1
  W_compressor/1 -> Mux/1
  W_throttle/1 -> Mux/2
  T_out_compressor/1 -> Mux/3
  T_out_IC_data/1 -> Mux/4

== system KD_cl_harness_forthao_breach/steps/Subsystem ==
  In1 : Inport
  Rate Limiter : RateLimiter  RisingSlewLimit=22  FallingSlewLimit=-22  SampleTimeMode=inherited  InitialCondition=30
  Unit Delay : UnitDelay  InitialCondition=30  SampleTime=-1
  Out1 : Outport
  wires:
  In1/1 -> Unit Delay/1
  Unit Delay/1 -> Rate Limiter/1
  Rate Limiter/1 -> Out1/1

== system KD_cl_harness_forthao_breach/steps/Subsystem1 ==
  In1 : Inport
  Rate Limiter : RateLimiter  RisingSlewLimit=1000  FallingSlewLimit=-1000  SampleTimeMode=inherited  InitialCondition=2500
  Unit Delay : UnitDelay  InitialCondition=2500  SampleTime=-1
  Out1 : Outport
  wires:
  Rate Limiter/1 -> Out1/1
  Unit Delay/1 -> Rate Limiter/1
  In1/1 -> Unit Delay/1

== system KD_cl_harness_forthao_breach/steps/Subsystem2 ==
  In1 : Inport
  Rate Limiter : RateLimiter  RisingSlewLimit=22  FallingSlewLimit=-22  SampleTimeMode=inherited  InitialCondition=5
  Unit Delay : UnitDelay  InitialCondition=5  SampleTime=-1
  Out1 : Outport
  wires:
  Rate Limiter/1 -> Out1/1
  Unit Delay/1 -> Rate Limiter/1
  In1/1 -> Unit Delay/1

== system KD_cl_harness_forthao_breach/EGR Throttle/EGR Throttle/Throttle Model2 ==
  TA[deg] : Inport
  Ne[rpm] : Inport  Port=2
  Pim[Pa] : Inport  Port=3
  Tim[K] : Inport  Port=4
  Pamb[Pa] : Inport  Port=5
  Tamb[K] : Inport  Port=6
  Air Model_map_use : Subsystem
  Ra : Constant  Value=const.Rair
  mt[kg/sec] : Outport
  forwardmt[kg/sec] : Outport  Port=2
  backwardmt[kg/sec] : Outport  Port=3
  wires:
  TA[deg]/1 -> Air Model_map_use/1(TA[deg])
  Pamb[Pa]/1 -> Air Model_map_use/5(Pa[Pa])
  Tamb[K]/1 -> Air Model_map_use/6(Ta[K])
  Pim[Pa]/1 -> Air Model_map_use/3(Pim[Pa])
  Tim[K]/1 -> Air Model_map_use/4(Tim[K])
  Air Model_map_use/1(mt[kg/sec]) -> mt[kg/sec]/1
  Ra/1 -> Air Model_map_use/7(R_im), Air Model_map_use/8(R_a)
  Air Model_map_use/2(forwardmt) -> forwardmt[kg/sec]/1
  Ne[rpm]/1 -> Air Model_map_use/2(Ne[rpm])
  Air Model_map_use/3(backwardmt) -> backwardmt[kg/sec]/1

== system KD_cl_harness_forthao_breach/EGR Valve/SVR EGR/EGR_model ==
  TA[deg] : Inport
  Ne[rpm] : Inport  Port=2
  Pim[Pa] : Inport  Port=3
  Tim[K] : Inport  Port=4
  Pamb[Pa] : Inport  Port=5
  Tamb[K] : Inport  Port=6
  Air Model_map_use : Subsystem
  Ra : Constant  Value=const.Rair
  mt[kg/sec] : Outport
  forwardmt[kg/sec] : Outport  Port=2
  wires:
  Ne[rpm]/1 -> Air Model_map_use/2(Ne[rpm])
  Air Model_map_use/2(forwardmt) -> forwardmt[kg/sec]/1
  Ra/1 -> Air Model_map_use/8(R_a), Air Model_map_use/7(R_im)
  Air Model_map_use/1(mt[kg/sec]) -> mt[kg/sec]/1
  Tim[K]/1 -> Air Model_map_use/4(Tim[K])
  Pim[Pa]/1 -> Air Model_map_use/3(Pim[Pa])
  Tamb[K]/1 -> Air Model_map_use/6(Ta[K])
  Pamb[Pa]/1 -> Air Model_map_use/5(Pa[Pa])
  TA[deg]/1 -> Air Model_map_use/1(TA[deg])

== system KD_cl_harness_forthao_breach/Exhaust Manifold/Exhaust Manifold/Cus_integrator ==
  in : Inport
  Integrator : Integrator  InitialCondition=IV.rho_exhaust_man  UpperSaturationLimit=maxL.rho_exhaust_man  LowerSaturationLimit=minL.rho_exhaust_man
  rho_exhaust : Outport
  wires:
  in/1 -> Integrator/1
  Integrator/1 -> rho_exhaust/1

== system KD_cl_harness_forthao_breach/Exhaust Manifold/Exhaust Manifold/Cus_integrator1 ==
  in : Inport
  Integrator1 : Integrator  InitialCondition=IV.F_exhaust  UpperSaturationLimit=maxL.F_exhuast_man  LowerSaturationLimit=minL.F_exhuast_man
  F2_exhaust : Outport
  wires:
  in/1 -> Integrator1/1
  Integrator1/1 -> F2_exhaust/1

== system KD_cl_harness_forthao_breach/Exhaust Manifold/Exhaust Manifold/Cus_integrator2 ==
  in : Inport
  Integrator2 : Integrator  InitialCondition=IV.p_exhaust_man  UpperSaturationLimit=maxL.p_exhaust_man  LowerSaturationLimit=minL.p_exhaust_man
  p_exhaust : Outport
  wires:
  Integrator2/1 -> p_exhaust/1
  in/1 -> Integrator2/1

== system KD_cl_harness_forthao_breach/Intake Manifold/Intake_manifold/Cus_integrator ==
  in : Inport
  Integrator : Integrator  InitialCondition=IV.rho_intake_man  UpperSaturationLimit=maxL.rho_intake_man  LowerSaturationLimit=minL.rho_intake_man
  rho_intake : Outport
  wires:
  in/1 -> Integrator/1
  Integrator/1 -> rho_intake/1

== system KD_cl_harness_forthao_breach/Intake Manifold/Intake_manifold/Cus_integrator1 ==
  in : Inport
  Integrator : Integrator  InitialCondition=IV.F_intake  UpperSaturationLimit="maxL.F1_intake_man   + 0.00001"  LowerSaturationLimit=minL.F1_intake_man
  F1_intake : Outport
  wires:
  in/1 -> Integrator/1
  Integrator/1 -> F1_intake/1

== system KD_cl_harness_forthao_breach/Intake Manifold/Intake_manifold/Cus_integrator2 ==
  in : Inport
  Integrator1 : Integrator  InitialCondition=IV.p_intake_man  UpperSaturationLimit=maxL.p_intake_man  LowerSaturationLimit=minL.p_intake_man
  p_intake : Outport
  wires:
  in/1 -> Integrator1/1
  Integrator1/1 -> p_intake/1

== system KD_cl_harness_forthao_breach/Turbo Rotational Dynamics/Turbo rot/Cus_integrator ==
  delta_torque : Inport
  Integrator1 : Integrator  InitialCondition=IV.omega_turbo_rads  UpperSaturationLimit=maxL.omega_turbo_rs  LowerSaturationLimit=minL.omega_turbo_rs
  NT_radS : Outport
  wires:
  delta_torque/1 -> Integrator1/1
  Integrator1/1 -> NT_radS/1

== system KD_cl_harness_forthao_breach/ctrl_rb_explicit_20131031_v2/EGR_max_flow/Air_Model_map_use ==
  Ne_rpm : Inport
  Pim_Pa : Inport  Port=2
  Pa_Pa : Inport  Port=3
  Ta_K : Inport  Port=4
  R_a : Inport  Port=5
  Forward_Flow : Subsystem
  Product1 : Product  Inputs=*//  SaturateOnIntegerOverflow=on  RndMeth=Zero  InputSameDT=on  OutDataTypeStr=Inherit: Same as first input
  Saturation : Saturate  UpperLimit=c_fflow_max  LowerLimit=c_fflow_min
      settings: AttributesFormatString=%<LowerLimit>\n%<UpperLimit>
  Saturation4 : Saturate  UpperLimit=c_ta_max  LowerLimit=c_ta_min
      settings: AttributesFormatString=%<LowerLimit>\n%<UpperLimit>
  mt_kg_per_sec : Outport
  wires:
  [Pa] -> Forward_Flow/3(Pa)
  Saturation/1 -> mt_kg_per_sec/1
  Ne_rpm/1 -> Forward_Flow/2(Ne_rpm)
  Forward_Flow/1(mt_dot_kg_per_s) -> Saturation/1
  [Ta] -> Saturation4/1
  [Pa] -> Product1/1
  [Ra] -> Product1/3
  R_a/1 -> [Ra]
  Ta_K/1 -> [Ta]
  Pa_Pa/1 -> [Pa]
  Pim_Pa/1 -> Forward_Flow/4(Pm)
  Product1/1 -> Forward_Flow/1(Ro_a)
  Saturation4/1 -> Product1/2

== system KD_cl_harness_forthao_breach/ctrl_rb_explicit_20131031_v2/PID/Filter1 ==
  Input : Inport
  Delay11 : Delay  DelayLength=1  InitialCondition=0
  Delay21 : Delay  DelayLength=1  InitialCondition=0
  SumA21 : Sum  Inputs=|+-  RndMeth=Nearest  SaturateOnIntegerOverflow=on  OutDataTypeStr=Inherit: Same as first input
      settings: AttributesFormatString=%<RndMeth>
  SumA31 : Sum  Inputs=|+-  RndMeth=Nearest  SaturateOnIntegerOverflow=on  OutDataTypeStr=Inherit: Same as first input
      settings: AttributesFormatString=%<RndMeth>
  SumB21 : Sum  Inputs=|++  RndMeth=Nearest  SaturateOnIntegerOverflow=on  OutDataTypeStr=Inherit: Same as first input
      settings: AttributesFormatString=%<RndMeth>
  SumB31 : Sum  Inputs=|++  RndMeth=Nearest  SaturateOnIntegerOverflow=on  OutDataTypeStr=Inherit: Same as first input
      settings: AttributesFormatString=%<RndMeth>
  a_2_1 : Gain  Gain=-1.5752583738614288  ParamDataTypeStr=float('double')  RndMeth=Nearest  SaturateOnIntegerOverflow=on  OutDataTypeStr=Inherit: Same as input
      settings: AttributesFormatString=%<Gain>\n%<RndMeth>
  a_3_1 : Gain  Gain=0.65083822277403669  ParamDataTypeStr=float('double')  RndMeth=Nearest  SaturateOnIntegerOverflow=on  OutDataTypeStr=Inherit: Same as input
      settings: AttributesFormatString=%<Gain>\n%<RndMeth>
  b_2_1 : Gain  Gain=2  ParamDataTypeStr=float('double')  RndMeth=Nearest  SaturateOnIntegerOverflow=on  OutDataTypeStr=Inherit: Same as input
      settings: AttributesFormatString=%<Gain>\n%<RndMeth>
  s_1 : Gain  Gain=0.018894962228151929  ParamDataTypeStr=float('double')  RndMeth=Nearest  SaturateOnIntegerOverflow=on  OutDataTypeStr=Inherit: Same as input
      settings: AttributesFormatString=%<Gain>\n%<RndMeth>
  Output : Outport
  wires:
  Delay21/1 -> SumB31/2, a_3_1/1
  a_3_1/1 -> SumA31/2
  b_2_1/1 -> SumB21/2
  Delay11/1 -> Delay21/1, b_2_1/1, a_2_1/1
  SumB31/1 -> Output/1
  SumB21/1 -> SumB31/1
  SumA31/1 -> Delay11/1, SumB21/1
  SumA21/1 -> SumA31/1
  s_1/1 -> SumA21/1
  Input/1 -> s_1/1
  a_2_1/1 -> [fb]
  [fb] -> SumA21/2

== system KD_cl_harness_forthao_breach/ctrl_rb_explicit_20131031_v2/PID/If_Action_Subsystem ==
  k : Inport
  Action Port : ActionPort  ActionType=then
  Gain6 : Gain  Gain=2
  Product1 : Product  Inputs=*/  RndMeth=Zero
  Saturation1 : Saturate  UpperLimit=inf  LowerLimit=0
      settings: AttributesFormatString=%<LowerLimit>\n%<UpperLimit>
  Saturation3 : Saturate  UpperLimit=c_inf  LowerLimit=c_p1e9
      settings: AttributesFormatString=%<LowerLimit>\n%<UpperLimit>
  Sum3 : Sum  Inputs=++|
  one : Constant  OutDataTypeStr=single  SampleTime=sample_time
      settings: AttributesFormatString=%<Value>\n%<SampleTime>
  Out : Outport
  wires:
  Saturation3/1 -> Product1/2
  Saturation1/1 -> Out/1
  Product1/1 -> Saturation1/1
  Gain6/1 -> Saturation3/1
  Sum3/1 -> Gain6/1
  one/1 -> Sum3/1
  [k] -> Sum3/2
  [k] -> Product1/1
  k/1 -> [k]

== system KD_cl_harness_forthao_breach/ctrl_rb_explicit_20131031_v2/PID/If_Action_Subsystem1 ==
  pin : Inport
  pex : Inport  Port=2
  k : Inport  Port=3
  Action Port : ActionPort  ActionType=else
  Product10 : Product  Inputs=**  RndMeth=Zero
  Product7 : Product  Inputs=*/  RndMeth=Zero
  Product8 : Product  Inputs=**  RndMeth=Zero
  Product9 : Product  Inputs=*//  RndMeth=Zero
  Saturation : Saturate  UpperLimit=inf  LowerLimit=0
      settings: AttributesFormatString=%<LowerLimit>\n%<UpperLimit>
  Saturation2 : Saturate  UpperLimit=c_inf  LowerLimit=c_p1e9
      settings: AttributesFormatString=%<LowerLimit>\n%<UpperLimit>
  Saturation4 : Saturate  UpperLimit=c_inf  LowerLimit=c_p1e9
      settings: AttributesFormatString=%<LowerLimit>\n%<UpperLimit>
  Sqrt1 : Sqrt  AlgorithmType=Newton-Raphson  SaturateOnIntegerOverflow=on
  Sum6 : Sum  Inputs=|+-
  Sum7 : Sum  Inputs=|+-
  Sum8 : Sum  Inputs=|++
  Sum9 : Sum  Inputs=|+-
  one3 : Constant  OutDataTypeStr=single  SampleTime=sample_time
      settings: AttributesFormatString=%<Value>\n%<SampleTime>
  one4 : Constant  OutDataTypeStr=single  SampleTime=sample_time
      settings: AttributesFormatString=%<Value>\n%<SampleTime>
  one5 : Constant  OutDataTypeStr=single  SampleTime=sample_time
      settings: AttributesFormatString=%<Value>\n%<SampleTime>
  two : Constant  Value=2  OutDataTypeStr=single  SampleTime=sample_time
      settings: AttributesFormatString=%<Value>\n%<SampleTime>
  Out : Outport
  wires:
  Saturation4/1 -> Product7/2
  Saturation2/1 -> Product9/3
  Saturation/1 -> Sqrt1/1
  Sqrt1/1 -> Out/1
  Product10/1 -> Saturation/1
  Sum8/1 -> Product10/1
  [pr] -> Sum9/2
  Sum9/1 -> Product10/2
  one5/1 -> Sum9/1
  [pr] -> Sum8/2
  Product9/1 -> Sum8/1
  [pr] -> Sum6/2
  Product7/1 -> [pr]
  [k] -> Saturation2/1
  two/1 -> Product9/2
  Product8/1 -> Product9/1
  Sum7/1 -> Product8/1
  Sum6/1 -> Product8/2
  one4/1 -> Sum7/2
  [k] -> Sum7/1
  [pex] -> Saturation4/1
  [pin] -> Product7/1
  one3/1 -> Sum6/1
  pin/1 -> [pin]
  k/1 -> [k]
  pex/1 -> [pex]

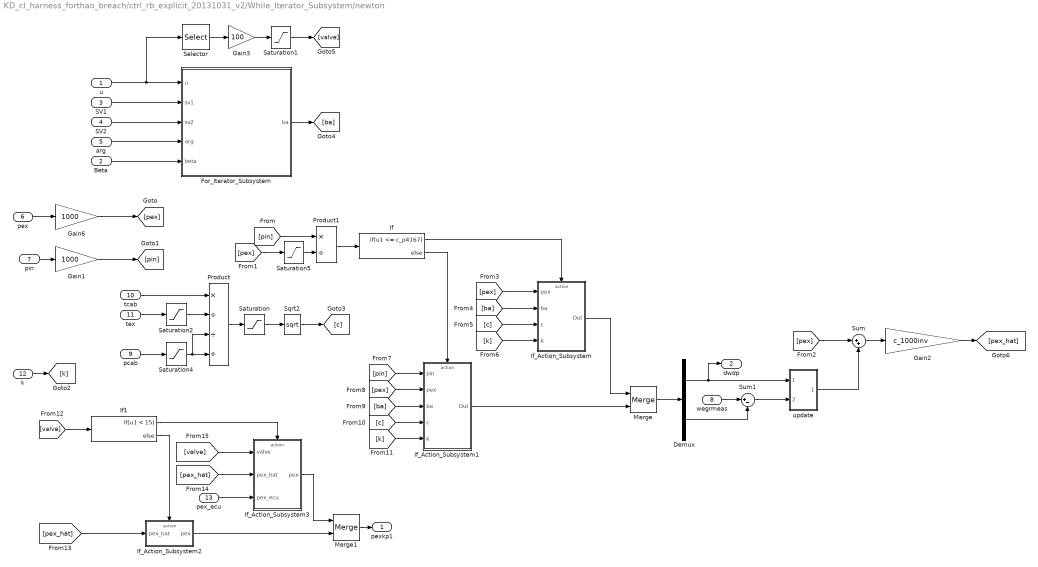
== system KD_cl_harness_forthao_breach/ctrl_rb_explicit_20131031_v2/While_Iterator_Subsystem/newton ==
  u : Inport
  Beta : Inport  Port=2
  SV1 : Inport  Port=3
  SV2 : Inport  Port=4
  arg : Inport  Port=5
  pex : Inport  Port=6
  pin : Inport  Port=7
  wegrmeas : Inport  Port=8
  pcab : Inport  Port=9
  tcab : Inport  Port=10
  tex : Inport  Port=11
  k : Inport  Port=12
  pex_ecu : Inport  Port=13
  Demux : Demux  Outputs=2
  For_Iterator_Subsystem : Subsystem  TreatAsAtomicUnit=on
  Gain1 : Gain  Gain=1000
      settings: AttributesFormatString=%<Gain>
  Gain2 : Gain  Gain=c_1000inv
      settings: AttributesFormatString=%<Gain>
  Gain3 : Gain  Gain=100
      settings: AttributesFormatString=%<Gain>
  Gain6 : Gain  Gain=1000
      settings: AttributesFormatString=%<Gain>
  If : If  IfExpression=u1 <= c_p4167
  If1 : If  IfExpression=u1 < 15
  If_Action_Subsystem : Subsystem  TreatAsAtomicUnit=on
  If_Action_Subsystem1 : Subsystem  TreatAsAtomicUnit=on
  If_Action_Subsystem2 : Subsystem  TreatAsAtomicUnit=on
  If_Action_Subsystem3 : Subsystem  TreatAsAtomicUnit=on
  Merge : Merge
  Merge1 : Merge
  Product : Product  Inputs=*///  RndMeth=Zero
  Product1 : Product  Inputs=*/  RndMeth=Zero
  Saturation : Saturate  UpperLimit=inf  LowerLimit=0
      settings: AttributesFormatString=%<LowerLimit>\n%<UpperLimit>
  Saturation1 : Saturate  UpperLimit=c_inf  LowerLimit=c_0
      settings: AttributesFormatString=%<LowerLimit>\n%<UpperLimit>
  Saturation2 : Saturate  UpperLimit=c_inf  LowerLimit=c_p1e9
      settings: AttributesFormatString=%<LowerLimit>\n%<UpperLimit>
  Saturation4 : Saturate  UpperLimit=c_inf  LowerLimit=c_p1e9
      settings: AttributesFormatString=%<LowerLimit>\n%<UpperLimit>
  Saturation5 : Saturate  UpperLimit=c_inf  LowerLimit=c_p1e9
      settings: AttributesFormatString=%<LowerLimit>\n%<UpperLimit>
  Selector : Selector  InputPortWidth=2
  Sqrt2 : Sqrt  AlgorithmType=Newton-Raphson  SaturateOnIntegerOverflow=on
  Sum : Sum  Inputs=|++
  Sum1 : Sum  Inputs=|+-
  update : Subsystem
  pexkp1 : Outport
  dwdp : Outport  Port=2
  wires:
  Saturation5/1 -> Product1/2
  Saturation4/1 -> Product/4, Product/3
  Saturation2/1 -> Product/2
  Saturation/1 -> Sqrt2/1
  Sum/1 -> Gain2/1
  update/1(delta) -> Sum/2
  [pex] -> Sum/1
  Merge/1 -> Demux/1
  If_Action_Subsystem1/1(Out) -> Merge/2
  If_Action_Subsystem/1(Out) -> Merge/1
  [k] -> If_Action_Subsystem1/5(k)
  [c] -> If_Action_Subsystem1/4(c)
  [ba] -> If_Action_Subsystem1/3(ba)
  [pex] -> If_Action_Subsystem1/2(pex)
  [pin] -> If_Action_Subsystem1/1(pin)
  If/2 -> If_Action_Subsystem1/Action
  [k] -> If_Action_Subsystem/4(k)
  [c] -> If_Action_Subsystem/3(c)
  [ba] -> If_Action_Subsystem/2(ba)
  [pex] -> If_Action_Subsystem/1(pex)
  If/1 -> If_Action_Subsystem/Action
  Product1/1 -> If/1
  [pex] -> Saturation5/1
  [pin] -> Product1/1
  For_Iterator_Subsystem/1(ba) -> [ba]
  Product/1 -> Saturation/1
  Gain1/1 -> [pin]
  Gain6/1 -> [pex]
  SV2/1 -> For_Iterator_Subsystem/3(sv2)
  k/1 -> [k]
  tex/1 -> Saturation2/1
  tcab/1 -> Product/1
  pcab/1 -> Saturation4/1
  wegrmeas/1 -> Sum1/1
  pin/1 -> Gain1/1
  pex/1 -> Gain6/1
  arg/1 -> For_Iterator_Subsystem/4(arg)
  SV1/1 -> For_Iterator_Subsystem/2(sv1)
  Beta/1 -> For_Iterator_Subsystem/5(beta)
  u/1 -> For_Iterator_Subsystem/1(u), Selector/1
  Demux/1 -> dwdp/1, update/1(dwdp)
  Demux/2 -> Sum1/2
  Sqrt2/1 -> [c]
  Selector/1 -> Gain3/1
  Gain3/1 -> Saturation1/1
  Saturation1/1 -> [valve]
  [valve] -> If1/1
  If1/2 -> If_Action_Subsystem2/Action
  If1/1 -> If_Action_Subsystem3/Action
  Gain2/1 -> [pex_hat]
  [pex_hat] -> If_Action_Subsystem2/1(pex_hat)
  [valve] -> If_Action_Subsystem3/1(valve)
  [pex_hat] -> If_Action_Subsystem3/2(pex_hat)
  pex_ecu/1 -> If_Action_Subsystem3/3(pex_ecu)
  If_Action_Subsystem2/1(pex) -> Merge1/2
  If_Action_Subsystem3/1(pex) -> Merge1/1
  Merge1/1 -> pexkp1/1
  Sum1/1 -> update/2(error)

== system KD_cl_harness_forthao_breach/ctrl_rb_explicit_20131031_v2/egr_est/custom_filter ==
  Input : Inport
  Data Store Read1 : DataStoreRead  DataStoreName=man_tuneFiltalpha  SampleTime=sample_time
  Data Store Read8 : DataStoreRead  DataStoreName=man_tuneFiltalpha  SampleTime=sample_time
  Delay1 : Delay  DelayLength=1  InitialCondition=0
  Product1 : Product  Inputs=**  RndMeth=Zero
  Product2 : Product  Inputs=**  RndMeth=Zero
  Saturation1 : Saturate  UpperLimit=1  LowerLimit=0
      settings: AttributesFormatString=%<LowerLimit>\n%<UpperLimit>
  Saturation4 : Saturate  UpperLimit=1  LowerLimit=0
      settings: AttributesFormatString=%<LowerLimit>\n%<UpperLimit>
  Sum1 : Sum  Inputs=+-|
  Sum11 : Sum  Inputs=++|
  man_tuneFiltalpha : Gain
  man_tuneFiltalpha1 : Gain
  zero1 : Constant  OutDataTypeStr=single  SampleTime=sample_time
      settings: AttributesFormatString=%<Value>\n%<SampleTime>
  Output : Outport  OutDataTypeStr=single
  wires:
  Input/1 -> Product1/2
  Delay1/1 -> Product2/1
  Data Store Read8/1 -> man_tuneFiltalpha1/1
  Product2/1 -> Sum11/1
  Sum1/1 -> Product1/1
  Data Store Read1/1 -> man_tuneFiltalpha/1
  Saturation4/1 -> Sum1/2
  Saturation1/1 -> Product2/2
  Product1/1 -> Sum11/2
  zero1/1 -> Sum1/1
  Sum11/1 -> Output/1, Delay1/1
  man_tuneFiltalpha/1 -> Saturation4/1
  man_tuneFiltalpha1/1 -> Saturation1/1

== system KD_cl_harness_forthao_breach/ctrl_rb_explicit_20131031_v2/egr_est/interp ==
  valve : Inport
  MAF : Inport  Port=2
  Wcyl : Inport  Port=3
  Product : Product  RndMeth=Zero
  Product1 : Product  RndMeth=Zero
  Sum : Sum  Inputs=-+|
  Sum1 : Sum  Inputs=++|
  interp : Lookup  InputValues=[0 15]  Table=[0 1]  LookUpMeth=Interpolation-Use End Values
      settings: AttributesFormatString=%<LookUpMeth>\n%<InputValues>
  one : Constant  OutDataTypeStr=single  SampleTime=sample_time
      settings: AttributesFormatString=%<Value>\n%<SampleTime>
  Wcylhat : Outport
  wires:
  valve/1 -> interp/1
  Wcyl/1 -> Product/1
  interp/1 -> Product/2, Sum/1
  one/1 -> Sum/2
  Sum/1 -> Product1/1
  MAF/1 -> Product1/2
  Product1/1 -> Sum1/2
  Product/1 -> Sum1/1
  Sum1/1 -> Wcylhat/1

== system KD_cl_harness_forthao_breach/ctrl_rb_explicit_20131031_v2/expcon/find_region ==
  u : Inport
  find_region : Subsystem  TreatAsAtomicUnit=on
  region_ic : Constant  Value=c_1_int  OutDataTypeStr=int32
      settings: AttributesFormatString=%<Value>
  region : Outport
  rv : Outport  Port=2
  wires:
  find_region/2(rv) -> rv/1
  find_region/1(region) -> region/1
  region_ic/1 -> find_region/2(IC)
  u/1 -> find_region/1(u)
